simulink model "svpwm_demo"  (R2022a)
settings: Solver=FixedStepAuto  StartTime=0.0  StopTime=50.0  FixedStep=0.01  RelTol=1e-3
settings Model: Creator=dxd36  LastModifiedBy=dxd36

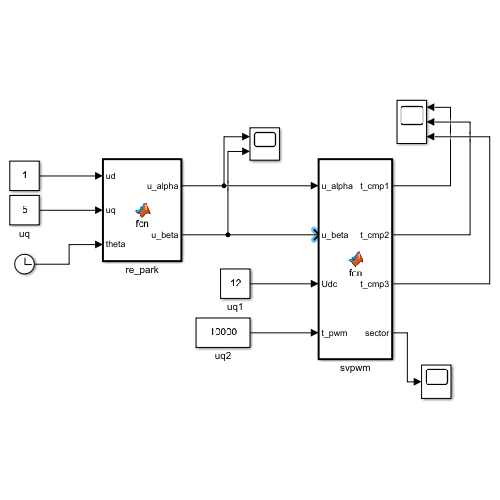
[thumbnail: Simulink's stored preview of the top-level diagram]
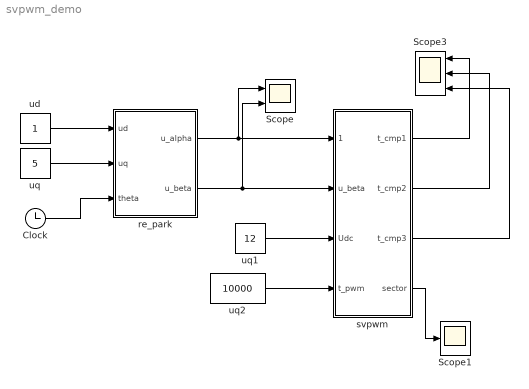
== system svpwm_demo ==
  Clock : Clock
      settings: Decimation=50
  Scope : Scope  NumInputPorts=2
  Scope1 : Scope
  Scope3 : Scope  NumInputPorts=3
  re_park : MATLAB Function  TreatAsAtomicUnit=on
  svpwm : MATLAB Function  TreatAsAtomicUnit=on
  ud : Constant
  uq : Constant  Value=5
  uq1 : Constant  Value=12
  uq2 : Constant  Value=10000
  wires:
  ud/1 -> re_park/1(ud)
  uq/1 -> re_park/2(uq)
  re_park/1(u_alpha) -> Scope/1, svpwm/1(u_alpha)
  re_park/2(u_beta) -> Scope/2, svpwm/2(u_beta)
  Clock/1 -> re_park/3(theta)
  svpwm/1(t_cmp1) -> Scope3/1
  svpwm/2(t_cmp2) -> Scope3/2
  svpwm/3(t_cmp3) -> Scope3/3
  svpwm/4(sector) -> Scope1/1
  uq1/1 -> svpwm/3(Udc)
  uq2/1 -> svpwm/4(t_pwm)

== matlab function svpwm_demo/svpwm ==
  data: u_alpha input; t_cmp1 output; u_beta input; Udc input; t_pwm input; t_cmp2 output; t_cmp3 output; sector output
function [t_cmp1, t_cmp2, t_cmp3, sector] = fcn(u_alpha, u_beta, Udc, t_pwm)

% 将其定义为单浮点精度的变量
t_cmp1 = double(0);
t_cmp2 = double(0);
t_cmp3 = double(0);
sector = single(0);

% step1: 自定义三个变量，用于判断扇区
v_ref1 = u_beta;
v_ref2 = (sqrt(3) * u_alpha - u_beta) / 2;
v_ref3 = (-sqrt(3) * u_alpha - u_beta) / 2;

% N = 4*C + 2*B + 1*A
% v_ref1 > 0 ---> A = 1
% v_ref2 > 0 ---> B = 1
% v_ref3 > 0 ---> C = 1
% 之所以用 if + end，就是为了系数的累加, 此处的 sector 并非是真正的扇区号，而是N值。
if (v_ref1 > 0)
    sector = single(1);
end

if (v_ref2 > 0)
    sector = sector + single(2);
end

if (v_ref3 > 0)
    sector = sector + single(4);
end

% step2: 依据不同的扇区来计算：T4、T6 的时间
% step2.1: 定义 X、Y、Z
tmp_k = sqrt(3) * t_pwm / Udc;
X = tmp_k * u_beta;
Y = tmp_k * (sqrt(3) * u_alpha + u_beta) / 2;
Z = tmp_k * (-sqrt(3) * u_alpha + u_beta) / 2;

% step2.2: Duty ratio calculation
switch (sector)   
    case 1
        T1 =  Z; T2 = Y; 
	case 2
        T1 =  Y; T2 = -X; 
	case 3
        T1 = -Z; T2 = X; 
	case 4
        T1 = -X; T2 = Z;
	case 5
        T1 =  X; T2 = -Y;
    otherwise
        T1 = -Y; T2 = -Z;
end

% step2.3:防止产生过调制
if T1 + T2 > t_pwm
    T1 = T1/(T1+T2);
    T2 = T2/(T1+T2);
end

ta = (t_pwm-(T1+T2)) / 4.0;
tb = ta+T1/2;
tc = tb+T2/2;

% step2.4: 计算比较器输出的值
switch (sector)
    case 1 
        t_cmp1=tb;
        t_cmp2=ta;
        t_cmp3=tc; 
        
    case 2 
        t_cmp1=ta;
        t_cmp2=tc;
        t_cmp3=tb; 
       
    case 3 
        t_cmp1=ta;
        t_cmp2=tb;
        t_cmp3=tc; 
        
    case 4 
        t_cmp1=tc;
        t_cmp2=tb;
        t_cmp3=ta;
        
    case 5 
        t_cmp1=tc;
        t_cmp2=ta;
        t_cmp3=tb;
        
   case 6
       t_cmp1=tb;
       t_cmp2=tc;
       t_cmp3=ta;
end
end

== matlab function svpwm_demo/re_park ==
  data: ud input; u_alpha output; uq input; u_beta output; theta input
function [u_alpha, u_beta] = fcn(ud, uq, theta)

u_alpha = ud * cos(theta) - uq * sin(theta);

u_beta  = uq * cos(theta) + ud * sin(theta);
